simulink model "EXP1_EX12"  (R2021b)
settings: Solver=VariableStepAuto  StartTime=0.0  StopTime=20  RelTol=1e-3
model workspace (MAT data in the model file):
  kp = [1  0; 0  1]
settings Model: LastModifiedBy=luang

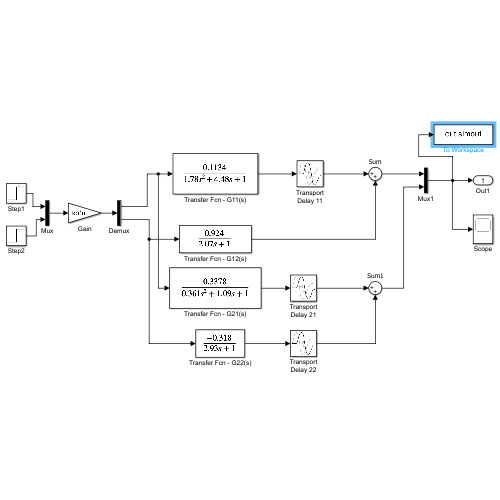
[thumbnail: Simulink's stored preview of the top-level diagram]
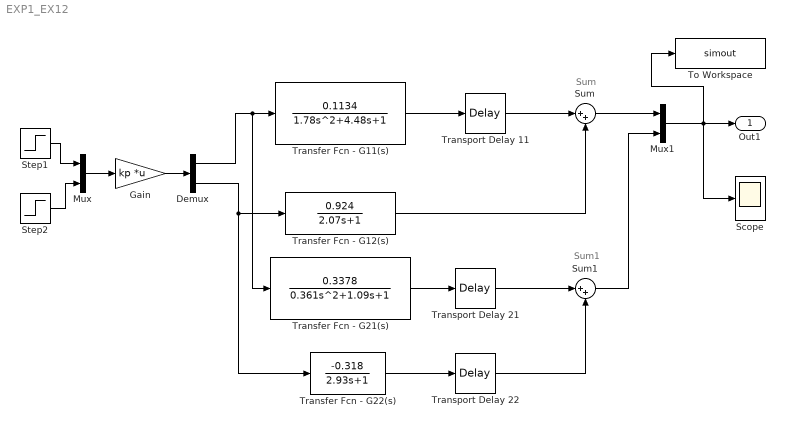
== system EXP1_EX12 ==
  note: Sum1
  note: Sum
  Demux : Demux  Outputs=2
  Gain : Gain  Gain=kp  Multiplication=Matrix(K*u)
  Mux : Mux  Inputs=2
  Mux1 : Mux  Inputs=2
  Scope : Scope
  Step1 : Step  SampleTime=0
  Step2 : Step  SampleTime=0
  Sum : Sum  Inputs=|++
  Sum1 : Sum  Inputs=|++
  To Workspace : ToWorkspace  VariableName=simout  SaveFormat=Structure With Time  SampleTime=-1
  Transfer Fcn - G11(s) : TransferFcn  Numerator=[0.1134]  Denominator=[1.78 4.48 1]  ContinuousStateAttributes='G11'
  Transfer Fcn - G12(s) : TransferFcn  Numerator=[0.924]  Denominator=[2.07 1]
  Transfer Fcn - G21(s) : TransferFcn  Numerator=[0.3378]  Denominator=[0.361 1.09 1]
  Transfer Fcn - G22(s) : TransferFcn  Numerator=[-0.318]  Denominator=[2.93 1]
  Transport Delay 11 : TransportDelay  DelayTime=0.72
  Transport Delay 21 : TransportDelay  DelayTime=0.3
  Transport Delay 22 : TransportDelay  DelayTime=1.29
  Out1 : Outport
  wires:
  Mux/1 -> Gain/1
  Transfer Fcn - G11(s)/1 -> Transport Delay 11/1
  Transport Delay 11/1 -> Sum/1
  Transfer Fcn - G12(s)/1 -> Sum/2
  Transfer Fcn - G21(s)/1 -> Transport Delay 21/1
  Transfer Fcn - G22(s)/1 -> Transport Delay 22/1
  Transport Delay 21/1 -> Sum1/1
  Transport Delay 22/1 -> Sum1/2
  Gain/1 -> Demux/1
  Step1/1 -> Mux/1
  Step2/1 -> Mux/2
  Sum/1 -> Mux1/1
  Sum1/1 -> Mux1/2
  Mux1/1 -> To Workspace/1, Scope/1, Out1/1
  Demux/1 -> Transfer Fcn - G21(s)/1, Transfer Fcn - G11(s)/1
  Demux/2 -> Transfer Fcn - G12(s)/1, Transfer Fcn - G22(s)/1
